simulink model "ex2_encoder"  (R2023b)
settings: Solver=FixedStepAuto  StartTime=0.0  StopTime=inf  FixedStep=Ts  RelTol=1e-3
InitFcn:
  | params
values from neighbouring files (symbols this model uses):
  den_Gd = Gd.Den{:}    [params.m]
  encoder_scale = 1/12/4 *2*pi    (= 0.1308996939)    [params.m]
  J = 0.02    [params.m]
  Kb = 0.1    [params.m]
  KD = 0.5    [params.m]
  Kf = 0.01    [params.m]
  KI = 0.1    [params.m]
  Km = 1    [params.m]
  KP = 0.7    [params.m]
  L = 0.5    [params.m]
  num_Gd = Gd.Num{:}    [params.m]
  R = 2.0    (= 2)    [params.m]
  Vlim = 12    [params.m]
  Wref = 100    [params.m]
libraries: simulink x1, arduinosensorlib x1, arduinolib x1
settings Model: SimulationMode=external  ExtModeTrigDuration=2  Creator=SJ  LastModifiedBy=tkdle
settings SolverCC: AutoInsertRateTranBlk=on
settings OptimizationCC: EnhancedBackFolding=on  PassReuseOutputArgsAs=Individual arguments  ZeroExternalMemoryAtStartup=off  ZeroInternalMemoryAtStartup=off  MaxStackSize=64  OptimizeBlockOrder=speed  DifferentSizesBufferReuse=on  OptimizationCustomize=off  EfficientTunableParamExpr=on
settings DebuggingCC: MultiTaskRateTransMsg=warning  ParameterTunabilityLossMsg=error
settings HardwareCC: ProdBitPerInt=16  ProdBitPerPointer=16  ProdBitPerSizeT=16  ProdBitPerPtrDiffT=16  ProdLargestAtomicFloat=None  ProdWordSize=8  ProdHWDeviceType=Atmel->AVR
settings SFSimCC: MATLABDynamicMemAlloc=off
settings RTWCC: Description=Embedded Coder  SystemTargetFile=ert.tlc  HardwareBoard=Arduino Mega 2560  TemplateMakefile=ert_default_tmf  Toolchain=Arduino AVR  BuildConfiguration=Faster Runs
settings CodeAppCC: ForceParamTrailComments=on  IgnoreCustomStorageClasses=off  OperatorAnnotations=on  SimulinkDataObjDesc=on  SFDataObjDesc=on  InsertBlockDesc=on
settings ERTTargetCC: SupportContinuousTime=on  SupportVariableSizeSignals=on  ExtMode=on  ExtModeTransport=3  ExtModeStaticAlloc=on  ExtModeAutomaticAllocSize=off  ExtModeStaticAllocSize=2048  ExtModeMexFile=ext_xcp  ExtModeMexArgs=0 3 921600  ExtModeIntrfLevel=Level2 - Open

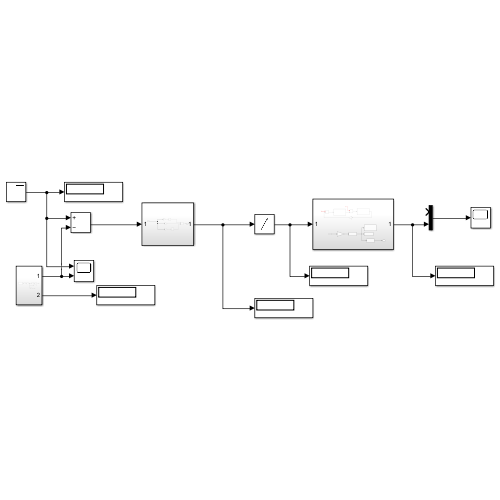
[thumbnail: Simulink's stored preview of the top-level diagram]
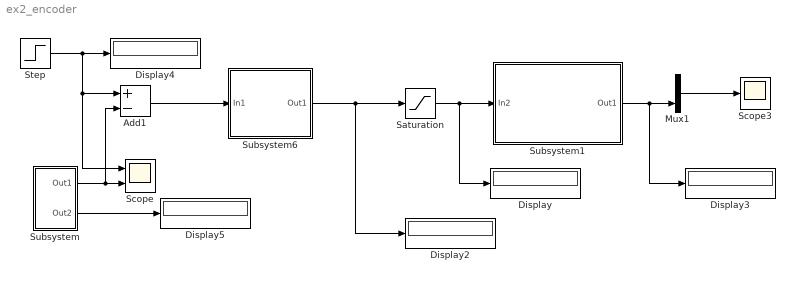
== system ex2_encoder ==
  Add1 : Sum  Inputs=+-
  Display{,2..5} (5 alike) : Display
  Mux1 : Mux  Inputs=2
  Saturation : Saturate  UpperLimit=12  LowerLimit=0
  Scope : Scope  NumInputPorts=2
  Scope3 : Scope
  Step : Step  After=Wref  SampleTime=0
  Subsystem : Subsystem
  Subsystem1 : Subsystem
  Subsystem6 : Subsystem
  wires:
  Subsystem/1(Out1) -> Add1/2, Scope/2
  Saturation/1 -> Subsystem1/1(In2), Display/1
  Mux1/1 -> Scope3/1
  Subsystem1/1(Out1) -> Display3/1, Mux1/2
  Subsystem/2(Out2) -> Display5/1
  Step/1 -> Scope/1, Add1/1, Display4/1
  Subsystem6/1(Out1) -> Display2/1, Saturation/1
  Add1/1 -> Subsystem6/1(In1)

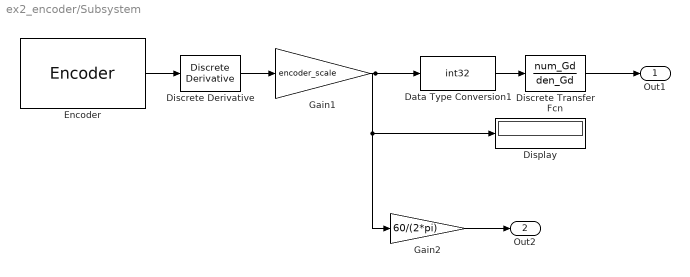
== system ex2_encoder/Subsystem ==
  Data Type Conversion1 : DataTypeConversion  OutDataTypeStr=int32  SaturateOnIntegerOverflow=off  RndMeth=Floor
  Discrete Transfer Fcn : DiscreteTransferFcn  Numerator=num_Gd  Denominator=den_Gd
  Discrete Derivative : simulink/Discrete/Discrete Derivative  gainval=1.0  ICPrevScaledInput=0.0  OutMin=[]  OutMax=[]  OutDataType=fixdt(1, 16)  OutScaling=2^-10  DoSatur=off
  Display : Display
  Encoder : arduinosensorlib/Encoder  InputA=20  InputB=21  Mode=No reset  SampleTime=-1
  Gain1 : Gain  Gain=encoder_scale
  Gain2 : Gain  Gain=60/(2*pi)
  Out1 : Outport
  Out2 : Outport  Port=2
  wires:
  Gain1/1 -> Display/1, Gain2/1, Data Type Conversion1/1
  Encoder/1 -> Discrete Derivative/1
  Gain2/1 -> Out2/1
  Data Type Conversion1/1 -> Discrete Transfer Fcn/1
  Discrete Derivative/1 -> Gain1/1
  Discrete Transfer Fcn/1 -> Out1/1

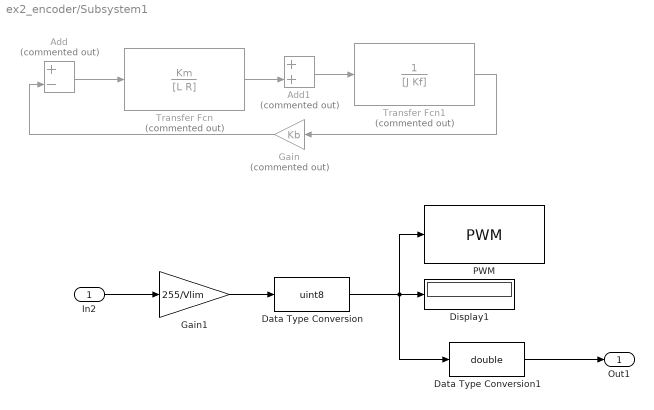
== system ex2_encoder/Subsystem1 ==
  In2 : Inport
  Add : Sum  Commented=on  Inputs=+-
  Add1 : Sum  Commented=on
  Data Type Conversion : DataTypeConversion  OutDataTypeStr=uint8  SaturateOnIntegerOverflow=off  RndMeth=Floor
  Data Type Conversion1 : DataTypeConversion  OutDataTypeStr=double  SaturateOnIntegerOverflow=off  RndMeth=Floor
  Display1 : Display
  Gain : Gain  Commented=on  Gain=Kb
  Gain1 : Gain  Gain=255/Vlim
  PWM : arduinolib/PWM  pinNumber=11  frequencyType=Default  desiredFrequency=490.2  achievableFrequency=490.2
  Transfer Fcn : TransferFcn  Commented=on  Numerator=Km  Denominator=[L R]
  Transfer Fcn1 : TransferFcn  Commented=on  Numerator=1  Denominator=[J Kf]
  Out1 : Outport
  wires:
  ? -> Add/1
  ? -> Add1/1
  Add/1 -> Transfer Fcn/1
  Add1/1 -> Transfer Fcn1/1
  Transfer Fcn/1 -> Add1/2
  Gain/1 -> Add/2
  Transfer Fcn1/1 -> Gain/1
  In2/1 -> Gain1/1
  Gain1/1 -> Data Type Conversion/1
  Data Type Conversion1/1 -> Out1/1
  Data Type Conversion/1 -> Data Type Conversion1/1, Display1/1, PWM/1

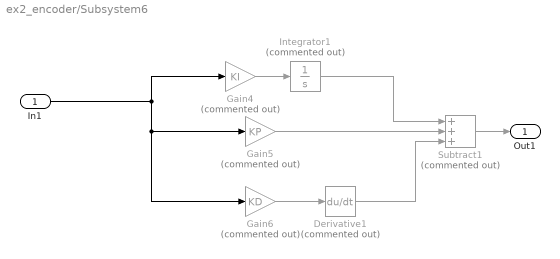
== system ex2_encoder/Subsystem6 ==
  In1 : Inport
  Derivative1 : Derivative  Commented=on
  Gain4 : Gain  Commented=on  Gain=KI
  Gain5 : Gain  Commented=on  Gain=KP
  Gain6 : Gain  Commented=on  Gain=KD
  Integrator1 : Integrator  Commented=on
  Subtract1 : Sum  Commented=on  Inputs=+++
  Out1 : Outport
  wires:
  Derivative1/1 -> Subtract1/3
  Gain4/1 -> Integrator1/1
  Integrator1/1 -> Subtract1/1
  Gain6/1 -> Derivative1/1
  Subtract1/1 -> Out1/1
  In1/1 -> Gain5/1, Gain6/1, Gain4/1
  Gain5/1 -> Subtract1/2
